simulink model "TRK_1b"  (R2026a)
settings: Solver=ode4  StopTime=1700  FixedStep=0.005
InitFcn:
  | TRK
values from neighbouring files (symbols this model uses):
  K_scheduled = zeros(length(V_op), 2)    [CAL3.m]    (also in CUB.m; DLC2.m; MUS.m; OHZ.m)
  V_op = 5:5:85    [CAL3.m]    (also in CUB.m; DLC2.m; MUS.m; OHZ.m)
  V_track = vx_scaled    [TRK.m]
  X_track = [linspace(0, runway_length, 200)'; runway_length + R_track * cos(theta_circ(2:end))]    [CAL3.m]    (also in CUB.m = [0; 5000]; DLC2.m = 0:0.1:total_track_length; MUS.m = [0; 2000]; OHZ.m = [0; 2000])
  Y_track = [zeros(200, 1); R_track + R_track * sin(theta_circ(2:end))]    [CAL3.m]    (also in CUB.m = [0; 0]; DLC2.m = zeros(size(X_track)); MUS.m = [0; 0]; OHZ.m = [0; 0])
undefined symbols (not defined in the file or in its folder): sim_params
libraries: sl_discontinuities x4, slpidlib x2, simulink x1
(part 3 of 3)

== matlab function TRK_1b/Vehicle Control Unit (VCU)/MATLAB Function ==
  settings: updateMethod=DISCRETE
  data: delta_curr input; pedal input; vx_curr input; vy_curr input; r_curr input; kappa_ref input; Fz_f_total input; Fz_r_total input; Fz_rl input; Fz_rr input; SOC input; T_batt input; T_motor input; V_op parameter; T_rr_motor_raw output size=1; K_scheduled parameter; T_rl_motor_raw output size=1; T_rr_fric output size=1; T_rl_fric output size=1; T_f_fric output size=1; Mz_cmd output size=1; r_ref output size=1; w_vec input
function [T_rr_motor_raw, T_rl_motor_raw, T_rr_fric, T_rl_fric, T_f_fric, Mz_cmd, r_ref] = vcu_allocator(delta_curr, pedal, vx_curr, vy_curr, r_curr, kappa_ref, Fz_f_total, Fz_r_total, Fz_rl, Fz_rr, SOC, T_batt, T_motor, V_op, K_scheduled, w_vec)
    
    % =========================================================================
    % 0. INITIALIZATION & PERSISTENT MEMORY FOR FILTER
    % =========================================================================
    persistent Mz_cmd_prev
    if isempty(Mz_cmd_prev)
        Mz_cmd_prev = 0.0;
    end

    % --- Force scalar numeric defaults for filter state and output ----
    Mz_cmd_prev = double(Mz_cmd_prev);  % ensure persistent is scalar double
    Mz_cmd = 0.0;                       % explicit scalar default for output
    Mz_cmd = double(Mz_cmd);

    T_rr_motor_raw = 0.0; T_rl_motor_raw = 0.0;
    T_rr_fric = 0.0; T_rl_fric = 0.0; T_f_fric = 0.0;
        
    T_rr_ideal = 0.0; 
    T_rl_ideal = 0.0;
    
    % Physical Constants
    Rw = 0.34; tw = 1.65; G = 10; mu_max = 1.2;
    
    % --- Per-Motor Limits ---
    P_motor_base = 250000; % 250 kW per motor
    T_motor_max = 400;     % 400 Nm per motor 
    T_fric_max_per_wheel = 3500;
    
    % =========================================================================
    % 1. BATTERY AND THERMAL DERATING
    % =========================================================================
    T_batt_cal = [-10, 0, 15, 45, 55, 60]; P_derate_batt_cal = [0, 0.5, 1.0, 1.0, 0.2, 0];
    T_motor_cal = [30, 90, 110, 130, 150]; P_derate_motor_cal = [1.0, 1.0, 1.0, 1.0, 1.0];
    SOC_vec = [0, 0.05, 0.15, 0.85, 0.95, 1.0]; 
    P_derate_SOC_dis = [0, 0.1, 1.0, 1.0, 1.0, 1.0]; P_derate_SOC_chg = [1.0, 1.0, 1.0, 1.0, 0.1, 0];
    
    derate_T_batt = interp1(T_batt_cal, P_derate_batt_cal, T_batt(1), 'linear', 0);
    derate_T_mot  = interp1(T_motor_cal, P_derate_motor_cal, T_motor(1), 'linear', 0);
    derate_T_total = min(derate_T_batt, derate_T_mot);
    
    derate_S_dis = interp1(SOC_vec, P_derate_SOC_dis, SOC(1), 'linear', 0);
    derate_S_chg = interp1(SOC_vec, P_derate_SOC_chg, SOC(1), 'linear', 0);
    
    P_avail_dis = P_motor_base * min(derate_T_total, derate_S_dis);
    P_avail_chg = P_motor_base * min(derate_T_total, derate_S_chg);
    
    vx_lqr = max(vx_curr(1), 5.0);
    
    % =========================================================================
    % 2. LQR TELEMETRY & COMMAND CALCULATION
    % =========================================================================
    vx_kmh = vx_curr(1) * 3.6;
    tv_blend_lower = 45.0; tv_blend_upper = 50.0; 
    if vx_kmh >= tv_blend_upper; tv_blend = 1.0;
    elseif vx_kmh <= tv_blend_lower; tv_blend = 0.0;
    else; tv_blend = (vx_kmh - tv_blend_lower) / (tv_blend_upper - tv_blend_lower); end
    
    K_dyn_1 = interp1(V_op, K_scheduled(:,1), vx_lqr, 'linear', 'extrap');
    K_dyn_2 = interp1(V_op, K_scheduled(:,2), vx_lqr, 'linear', 'extrap');
             
    L = 2.6; K_us = 0.002; 
    r_ref_raw = (vx_lqr * delta_curr(1)) / (L * (1 + K_us * vx_lqr^2));
    r_max_phys = (mu_max * 9.81 * 0.95) / vx_lqr; 
    r_ref = max(-r_max_phys, min(r_max_phys, r_ref_raw));
    
    % LQR Output (Raw, high-frequency request)
    Mz_req_raw = tv_blend * -(K_dyn_1(1) * vy_curr(1) + K_dyn_2(1) * (r_curr(1) - r_ref));
    Mz_cmd_raw = max(-2500, min(2500, Mz_req_raw)); 
    
    % --- DISCRETE FIRST-ORDER LOW-PASS FILTER ---
    % Filters out commands faster than the hydraulic brakes can physically respond to.
    dt = 0.001; % Assuming a 1ms fixed-step solver
    tau = 0;  % 0.5s time constant (blocks frequencies above ~2 rad/s)
    alpha = dt / (tau + dt); % Exponential smoothing factor
    
    % Ensure scalars and numeric type before filtering
    Mz_cmd_raw = double(Mz_cmd_raw);
    Mz_cmd_prev = double(Mz_cmd_prev);
    
    Mz_cmd = (1 - alpha) * Mz_cmd_prev + alpha * Mz_cmd_raw;
    Mz_cmd = double(Mz_cmd); % enforce scalar numeric
    Mz_cmd_prev = Mz_cmd; % Save state for the next solver step
    % --------------------------------------------

    % Convert Yaw Moment to Wheel Torque Delta
    T_delta_wheel = (Mz_cmd * Rw) / tw;
    
    % =========================================================================
    % 3. DYNAMIC MOTOR POWER LIMITS
    % =========================================================================
    w_motor_rl = max(abs(w_vec(3) * G), 0.1); 
    w_motor_rr = max(abs(w_vec(4) * G), 0.1); 
    
    T_limit_rl_dis = P_avail_dis / ((1)*w_motor_rl); T_limit_rr_dis = P_avail_dis / ((1)*w_motor_rr);
    T_motor_lim_rl_dis = min(T_motor_max, T_limit_rl_dis); T_motor_lim_rr_dis = min(T_motor_max, T_limit_rr_dis);
    T_motor_lim_rl_chg = max(-T_motor_max, -(P_avail_chg / ((1)*w_motor_rl)));
    T_motor_lim_rr_chg = max(-T_motor_max, -(P_avail_chg / ((1)*w_motor_rr)));
    
    % =========================================================================
    % 4. TORQUE ALLOCATION: DRIVE VS BRAKE
    % =========================================================================
    if pedal(1) >= 0
        % --- DRIVE MODE: LQR BRAKE VECTORING WITH OPEN DIFF ---
        
        T_req_total_motor = pedal(1) * (T_motor_lim_rl_dis + T_motor_lim_rr_dis); 
        
        v_hub_rl = max(vx_curr(1) - (tw/2)*r_curr(1), 1.0);
        v_hub_rr = max(vx_curr(1) + (tw/2)*r_curr(1), 1.0);
        
        kappa_rl = (w_vec(3)*Rw - v_hub_rl) / v_hub_rl;
        kappa_rr = (w_vec(4)*Rw - v_hub_rr) / v_hub_rr;
        
        % ---------------------------------------------------------------------
        % TIER 1: AXLE-LEVEL MOTOR TCS
        % ---------------------------------------------------------------------
        worst_kappa_rear = max(kappa_rl, kappa_rr);
        motor_slip_target = 0.10; 
        
        vx_threshold = 15 / 3.6; 
        if vx_curr(1) < vx_threshold; active_Kp = 100 * (vx_curr(1) / vx_threshold);
        else; active_Kp = 1000; end
        
        if worst_kappa_rear > motor_slip_target
            T_req_total_motor = max(0, T_req_total_motor - active_Kp * (worst_kappa_rear - motor_slip_target));
        end
        
        % ---------------------------------------------------------------------
        % TIER 2: LQR BRAKE VECTORING
        % ---------------------------------------------------------------------
        T_base_motor = T_req_total_motor / 2.0;
        T_delta_motor = T_delta_wheel / G;
        
        if Mz_cmd >= 0 % LEFT TURN (Right wheel needs more torque)
            T_mot_req_raw = T_base_motor + abs(T_delta_motor);
            T_rr_ideal = min(T_motor_lim_rr_dis, T_mot_req_raw);
            T_rl_ideal = min(T_motor_lim_rl_dis, T_mot_req_raw);
            
            T_rl_req_wheel = (T_base_motor - abs(T_delta_motor)) * G;
            T_rl_fric = max(-T_fric_max_per_wheel, T_rl_req_wheel - (T_rl_ideal * G));
            T_rr_fric = 0.0;
            
        else % RIGHT TURN (Left wheel needs more torque)
            T_mot_req_raw = T_base_motor + abs(T_delta_motor);
            T_rl_ideal = min(T_motor_lim_rl_dis, T_mot_req_raw);
            T_rr_ideal = min(T_motor_lim_rr_dis, T_mot_req_raw);
            
            T_rr_req_wheel = (T_base_motor - abs(T_delta_motor)) * G;
            T_rr_fric = max(-T_fric_max_per_wheel, T_rr_req_wheel - (T_rr_ideal * G));
            T_rl_fric = 0.0;
        end
        
    else
        % --- BRAKE MODE: LQR VECTORING + REGEN + ABS ---
        bias_f = 0.70;
        total_grip_cap_wheel = mu_max * (Fz_f_total(1) + Fz_r_total(1)) * Rw * 0.90;
        T_req_total_wheel = pedal(1) * total_grip_cap_wheel; 
        
        T_f_fric = max(-mu_max * Fz_f_total(1) * Rw * 0.90, T_req_total_wheel * bias_f);
        
        T_base_rr_wheel = (T_req_total_wheel * (1 - bias_f) * 0.5) + T_delta_wheel;
        T_base_rl_wheel = (T_req_total_wheel * (1 - bias_f) * 0.5) - T_delta_wheel;
        
        v_hub_fl = max(vx_curr(1) - (tw/2)*r_curr(1), 1.0); v_hub_fr = max(vx_curr(1) + (tw/2)*r_curr(1), 1.0);
        v_hub_rl = max(vx_curr(1) - (tw/2)*r_curr(1), 1.0); v_hub_rr = max(vx_curr(1) + (tw/2)*r_curr(1), 1.0);
        
        kappa_fl = (w_vec(1)*Rw - v_hub_fl) / v_hub_fl; kappa_fr = (w_vec(2)*Rw - v_hub_fr) / v_hub_fr;
        kappa_rl = (w_vec(3)*Rw - v_hub_rl) / v_hub_rl; kappa_rr = (w_vec(4)*Rw - v_hub_rr) / v_hub_rr;
        
        slip_limit_abs = -0.10; Kp_abs = 5000;
        
        if min(kappa_fl, kappa_fr) < slip_limit_abs
            T_f_fric = min(0, T_f_fric - Kp_abs * (min(kappa_fl, kappa_fr) - slip_limit_abs));
        end
        
        T_rl_abs_wheel = T_base_rl_wheel;
        T_rr_abs_wheel = T_base_rr_wheel;
        if kappa_rl < slip_limit_abs
            T_rl_abs_wheel = min(0, T_rl_abs_wheel - Kp_abs * (kappa_rl - slip_limit_abs));
        end
        if kappa_rr < slip_limit_abs
            T_rr_abs_wheel = min(0, T_rr_abs_wheel - Kp_abs * (kappa_rr - slip_limit_abs));
        end
        
        T_rl_ideal = max(T_motor_lim_rl_chg, T_rl_abs_wheel / G);
        T_rr_ideal = max(T_motor_lim_rr_chg, T_rr_abs_wheel / G);
        
        T_rl_fric = max(-T_fric_max_per_wheel, min(0, T_rl_abs_wheel - (T_rl_ideal * G)));
        T_rr_fric = max(-T_fric_max_per_wheel, min(0, T_rr_abs_wheel - (T_rr_ideal * G)));
    end
    
    if vx_curr(1) < 1.5
        T_rr_motor_raw = 0.0; T_rl_motor_raw = 0.0;
        T_f_fric = 0.0; T_rr_fric = 0.0; T_rl_fric = 0.0;
    else
        T_rr_motor_raw = T_rr_ideal;
        T_rl_motor_raw = T_rl_ideal;
    end

    % --- Ensure Mz_cmd is a scalar double on output --------------------
    Mz_cmd = double(Mz_cmd);
    if numel(Mz_cmd) ~= 1
        Mz_cmd = Mz_cmd(1);   % reduce to scalar if accidentally vector
    end
end

== matlab function TRK_1b/Vehicle & Powertrain Plant1/MATLAB Function ==
  data: delta input; Trr_m input; Trl_m input; Trr_f input; Trl_f input; Tf_f input; vx input; vy input; r input; psi input; SOC input; T_batt input; T_motor input; w_fl input; w_fr input; w_rl input; w_rr input; mu_left input; mu_right input; vx_dot output; vy_dot output; r_dot output; X_dot output; Y_dot output; psi_dot output; s_dot output; SOC_dot output; T_batt_dot output; T_mot_dot output; Fz_f_tot output; Fz_r_tot output; Fz_rl output; Fz_rr output; Fx_vec output; Fy_vec output; Fz_vec output; w_vec output; w_dot_vec output; veh_params parameter; I_batt output; Pwr_Elec output
function [vx_dot, vy_dot, r_dot, X_dot, Y_dot, psi_dot, s_dot, SOC_dot, T_batt_dot, T_mot_dot, Fz_f_tot, Fz_r_tot, Fz_rl, Fz_rr, Fx_vec, Fy_vec, Fz_vec, w_vec, w_dot_vec, I_batt, Pwr_Elec] = vehicle_physics_engine_mus(delta, Trr_m, Trl_m, Trr_f, Trl_f, Tf_f, vx, vy, r, psi, SOC, T_batt, T_motor, w_fl, w_fr, w_rl, w_rr, mu_left, mu_right, veh_params)
    
    % =========================================================================
    % 0. EXPLICIT OUTPUT INITIALIZATION & SCALAR COERCION 
    % =========================================================================
    vx_dot = 0.0; vy_dot = 0.0; r_dot = 0.0; 
    X_dot = 0.0; Y_dot = 0.0; psi_dot = 0.0; s_dot = 0.0;
    SOC_dot = 0.0; T_batt_dot = 0.0; T_mot_dot = 0.0;
    Fz_f_tot = 0.0; Fz_r_tot = 0.0; Fz_rl = 0.0; Fz_rr = 0.0;
    Fx_vec = zeros(1,4); Fy_vec = zeros(1,4); Fz_vec = zeros(1,4);
    w_vec = zeros(1,4); w_dot_vec = zeros(1,4);
    I_batt = 0.0; 
    Pwr_Elec = 0.0; 

    % Force scalar inputs
    delta = delta(1); vx = vx(1); vy = vy(1); r = r(1); psi = psi(1);
    Trr_m = Trr_m(1); Trl_m = Trl_m(1); Trr_f = Trr_f(1); Trl_f = Trl_f(1); Tf_f = Tf_f(1);
    SOC = SOC(1); T_batt = T_batt(1); T_motor = T_motor(1);
    w_fl = w_fl(1); w_fr = w_fr(1); w_rl = w_rl(1); w_rr = w_rr(1);
    mu_left = mu_left(1); mu_right = mu_right(1); % NEW DYNAMIC FRICTION INPUTS

    % =========================================================================
    % HIGH-FIDELITY EV VEHICLE DYNAMICS PLANT MODEL
    % =========================================================================
    
    % ---------------------------------------------------------------------
    % 1. UNPACK CENTRALIZED PARAMETERS
    % ---------------------------------------------------------------------
    m = veh_params.m(1); Iz = veh_params.Iz(1); lf = veh_params.lf(1); lr = veh_params.lr(1); L = veh_params.L(1);
    tw = veh_params.tw(1); h_cg = veh_params.h_cg(1); Rw = veh_params.Rw(1); Iw = veh_params.Iw(1); 
    G = veh_params.G(1); g = veh_params.g(1); rho = veh_params.rho(1); CdA = veh_params.CdA(1);
    roll_bias_f = veh_params.roll_bias_f(1); 
    
    C_rr = veh_params.C_rr(1);
    ks_f = veh_params.ks_f(1)/2; ks_r = veh_params.ks_r(1)/2;
    C_tire = veh_params.C_tire(1); E_tire = veh_params.E_tire(1);
    
    if abs(vx) < 0.5
        vx_safe = 0.5 * sign(vx + 1e-6); 
    else
        vx_safe = vx;
    end
    
    F_aero_drag = 0.5 * rho * CdA * vx_safe * abs(vx_safe);
    
    % ---------------------------------------------------------------------
    % 2. INDEPENDENT TIRE PEAK CALIBRATION (UPDATED FOR MU-SPLIT)
    % ---------------------------------------------------------------------
    Fz_axle_f_static = m * g * (lr / L); 
    Fz_axle_r_static = m * g * (lf / L); 
    
    % Calculate peak loads (D) based on local friction
    D_tire_fl = mu_left * (Fz_axle_f_static / 2); 
    D_tire_fr = mu_right * (Fz_axle_f_static / 2); 
    D_tire_rl = mu_left * (Fz_axle_r_static / 2); 
    D_tire_rr = mu_right * (Fz_axle_r_static / 2); 
    
    % Calculate stiffness factors (B) individually 
    B_tire_fl = ks_f / (C_tire * max(D_tire_fl, 1e-6) * 2); 
    B_tire_fr = ks_f / (C_tire * max(D_tire_fr, 1e-6) * 2); 
    B_tire_rl = ks_r / (C_tire * max(D_tire_rl, 1e-6) * 2); 
    B_tire_rr = ks_r / (C_tire * max(D_tire_rr, 1e-6) * 2); 
    
    % ---------------------------------------------------------------------
    % 3. 3D WEIGHT TRANSFER 
    % ---------------------------------------------------------------------
    Trr_tot = Trr_m * G + Trr_f;
    Trl_tot = Trl_m * G + Trl_f;
    Tf_tot_half = Tf_f / 2; 
    
    Fx_fl_tq = Tf_tot_half / Rw; Fx_fr_tq = Tf_tot_half / Rw;
    Fx_rl_tq = Trl_tot / Rw; Fx_rr_tq = Trr_tot / Rw;
    
    ax_est = ((Fx_fl_tq + Fx_fr_tq + Fx_rl_tq + Fx_rr_tq) - F_aero_drag) / m;
    ay_est = vx_safe * r;
    
    Fz_f_tot = m * g * (lr / L) - m * ax_est * (h_cg / L);
    Fz_r_tot = m * g * (lf / L) + m * ax_est * (h_cg / L);
    
    dFz_y_f = m * ay_est * (h_cg / tw) * roll_bias_f;
    dFz_y_r = m * ay_est * (h_cg / tw) * (1 - roll_bias_f);
    
    Fz_max_f = Fz_axle_f_static * 2.5; 
    Fz_max_r = Fz_axle_r_static * 2.5;
    
    Fz_fl = max(100, min(Fz_max_f, Fz_f_tot / 2 - dFz_y_f));
    Fz_fr = max(100, min(Fz_max_f, Fz_f_tot / 2 + dFz_y_f));
    Fz_rl = max(100, min(Fz_max_r, Fz_r_tot / 2 - dFz_y_r));
    Fz_rr = max(100, min(Fz_max_r, Fz_r_tot / 2 + dFz_y_r));
    Fz_vec = [Fz_fl, Fz_fr, Fz_rl, Fz_rr];
    
    % ---------------------------------------------------------------------
    % 4. VECTOR-SUM PACEJKA COMBINED SLIP MODEL (UPDATED FOR MU-SPLIT)
    % ---------------------------------------------------------------------
    v_hub_fl = vx_safe - (tw / 2) * r; v_hub_fr = vx_safe + (tw / 2) * r;
    v_hub_rl = vx_safe - (tw / 2) * r; v_hub_rr = vx_safe + (tw / 2) * r;
    
    k_fl = (w_fl * Rw - v_hub_fl) / max(abs(v_hub_fl), 1.0);
    k_fr = (w_fr * Rw - v_hub_fr) / max(abs(v_hub_fr), 1.0);
    k_rl = (w_rl * Rw - v_hub_rl) / max(abs(v_hub_rl), 1.0);
    k_rr = (w_rr * Rw - v_hub_rr) / max(abs(v_hub_rr), 1.0);
    
    alpha_fl = delta - atan((vy + lf * r) / max(abs(v_hub_fl), 1.0));
    alpha_fr = delta - atan((vy + lf * r) / max(abs(v_hub_fr), 1.0));
    alpha_rl = -atan((vy - lr * r) / max(abs(v_hub_rl), 1.0));
    alpha_rr = -atan((vy - lr * r) / max(abs(v_hub_rr), 1.0));
    
    sigma_fl = sqrt(k_fl^2 + tan(alpha_fl)^2) + 1e-6;
    sigma_fr = sqrt(k_fr^2 + tan(alpha_fr)^2) + 1e-6;
    sigma_rl = sqrt(k_rl^2 + tan(alpha_rl)^2) + 1e-6;
    sigma_rr = sqrt(k_rr^2 + tan(alpha_rr)^2) + 1e-6;
    
    F_tot_fl = mu_left * Fz_fl * sin(C_tire * atan(B_tire_fl * sigma_fl - E_tire * (B_tire_fl * sigma_fl - atan(B_tire_fl * sigma_fl))));
    F_tot_fr = mu_right * Fz_fr * sin(C_tire * atan(B_tire_fr * sigma_fr - E_tire * (B_tire_fr * sigma_fr - atan(B_tire_fr * sigma_fr))));
    F_tot_rl = mu_left * Fz_rl * sin(C_tire * atan(B_tire_rl * sigma_rl - E_tire * (B_tire_rl * sigma_rl - atan(B_tire_rl * sigma_rl))));
    F_tot_rr = mu_right * Fz_rr * sin(C_tire * atan(B_tire_rr * sigma_rr - E_tire * (B_tire_rr * sigma_rr - atan(B_tire_rr * sigma_rr))));
    
    Fx_fl = F_tot_fl * (k_fl / sigma_fl) - C_rr * Fz_fl * tanh(v_hub_fl * 10);
    Fx_fr = F_tot_fr * (k_fr / sigma_fr) - C_rr * Fz_fr * tanh(v_hub_fr * 10);
    Fx_rl = F_tot_rl * (k_rl / sigma_rl) - C_rr * Fz_rl * tanh(v_hub_rl * 10);
    Fx_rr = F_tot_rr * (k_rr / sigma_rr) - C_rr * Fz_rr * tanh(v_hub_rr * 10);
    Fx_vec = [Fx_fl, Fx_fr, Fx_rl, Fx_rr];
    
    Fy_fl = F_tot_fl * (tan(alpha_fl) / sigma_fl);
    Fy_fr = F_tot_fr * (tan(alpha_fr) / sigma_fr);
    Fy_rl = F_tot_rl * (tan(alpha_rl) / sigma_rl);
    Fy_rr = F_tot_rr * (tan(alpha_rr) / sigma_rr);
    Fy_vec = [Fy_fl, Fy_fr, Fy_rl, Fy_rr];
    
    % ---------------------------------------------------------------------
    % 5. CHASSIS & WHEEL INTEGRATORS
    % ---------------------------------------------------------------------
    w_fl_dot = (-abs(Tf_f / 2) * sign(w_fl) - Fx_fl * Rw) / Iw;
    w_fr_dot = (-abs(Tf_f / 2) * sign(w_fr) - Fx_fr * Rw) / Iw;
    w_rl_dot = (Trl_m * G - abs(Trl_f) * sign(w_rl) - Fx_rl * Rw) / Iw;
    w_rr_dot = (Trr_m * G - abs(Trr_f) * sign(w_rr) - Fx_rr * Rw) / Iw;
    w_dot_vec = [w_fl_dot, w_fr_dot, w_rl_dot, w_rr_dot];
    w_vec = [w_fl, w_fr, w_rl, w_rr];
    
    sum_Fx = (Fx_fl + Fx_fr) * cos(delta) - (Fy_fl + Fy_fr) * sin(delta) + Fx_rl + Fx_rr;
    vx_dot = (sum_Fx - F_aero_drag) / m + vy * r;
    
    sum_Fy = (Fy_fl + Fy_fr) * cos(delta) + (Fx_fl + Fx_fr) * sin(delta) + Fy_rl + Fy_rr;
    vy_dot = sum_Fy / m - vx_safe * r;
    
    M_front = lf * ((Fy_fl + Fy_fr) * cos(delta) + (Fx_fl + Fx_fr) * sin(delta));
    M_rear  = -lr * (Fy_rl + Fy_rr);
    M_tv    = (Fx_rr - Fx_rl) * (tw / 2); 
    r_dot  = (M_front + M_rear + M_tv) / Iz;
    
    X_dot   = vx_safe * cos(psi) - vy * sin(psi);
    Y_dot   = vx_safe * sin(psi) + vy * cos(psi);
    psi_dot = r;
    s_dot   = vx_safe;
    
    % ---------------------------------------------------------------------
    % 6. THERMALS & SOC (R-INT BATTERY MODEL)
    % ---------------------------------------------------------------------
    P_mech = (Trr_m + Trl_m) * G * (vx_safe / Rw);
    P_elec = P_mech; 
    
    if P_mech > 500
        P_elec = P_mech / 0.90; 
    elseif P_mech < -500
        P_elec = P_mech * 0.90; 
    end
    
    V_oc = veh_params.V_pack; 
    R_int = 0.015;            
    
    discriminant = V_oc^2 - 4 * R_int * P_elec;
    if discriminant < 0; discriminant = 0; end
    
    I_curr = (V_oc - sqrt(discriminant)) / (2 * R_int);
    I_batt = I_curr; Pwr_Elec = P_elec;
    
    SOC_dot = -I_curr / (veh_params.Cap_Ah * 3600);
    T_batt_dot = ((I_curr^2) * R_int - veh_params.hA_cool_batt * (T_batt - veh_params.T_coolant_batt)) / (veh_params.m_batt * veh_params.cp_batt);
    T_mot_dot  = (abs(P_elec - P_mech) - veh_params.hA_cool_motor * (T_motor - veh_params.T_ambient)) / (veh_params.m_motor * veh_params.cp_motor);
end
